simulink model "class_d_ff"  (R2024b)
settings: Solver=VariableStepAuto  StartTime=0.0  StopTime=5e-3  MaxStep=1e-8  RelTol=1e-9
undefined symbols (not defined in the file): gaussian
libraries: simulink x2
settings Model: SimulationMode=rapid-accelerator  Creator=Aaron  LastModifiedBy=Aaron
settings SolverCC: ShapePreserveControl=EnableAll  ZeroCrossAlgorithm=Adaptive

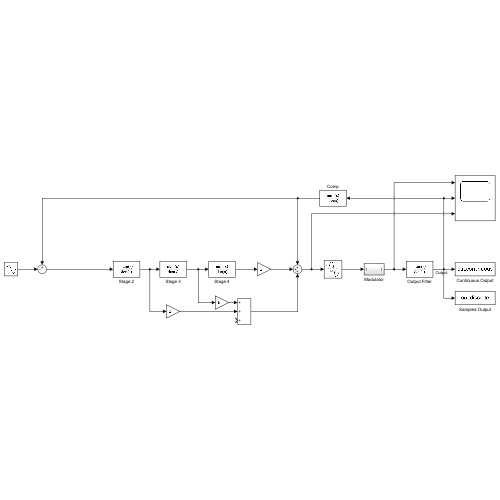
[thumbnail: Simulink's stored preview of the top-level diagram]
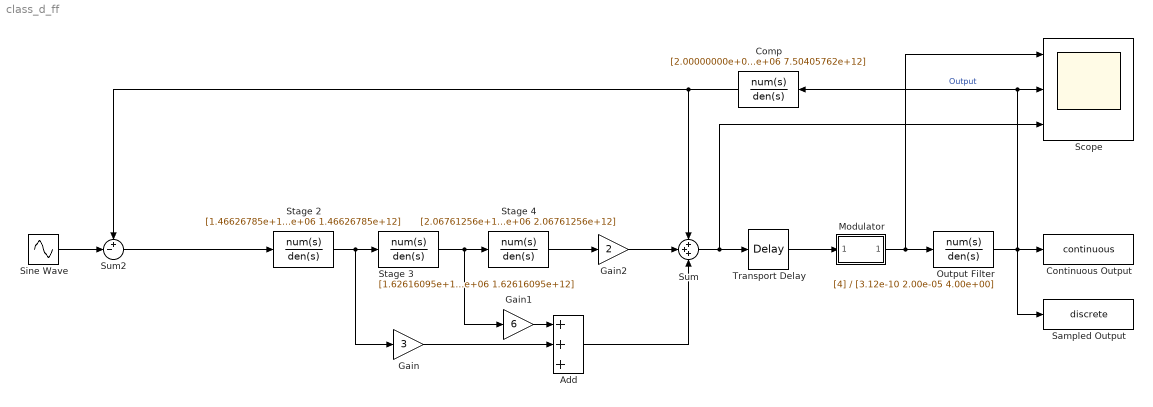
== system class_d_ff ==
  Add : Sum  Inputs=+++
  Comp : TransferFcn  Numerator=[2.00000000e+00 6.03185789e+06 4.54791371e+12]  Denominator=[1.00000000e+00 5.57946855e+06 7.50405762e+12]
  Continuous Output : ToWorkspace  VariableName=continuous  SaveFormat=Structure With Time  SampleTime=-1
  Gain : Gain  Gain=3
  Gain1 : Gain  Gain=6
  Gain2 : Gain  Gain=2
  Modulator : Subsystem
  Output Filter : TransferFcn  Numerator=[4]  Denominator=[3.12e-10 2.00e-05 4.00e+00]
  Sampled Output : ToWorkspace  VariableName=discrete  SampleTime=-1
  Scope : Scope  NumInputPorts=3
  Sine Wave : Sin  Amplitude=8  Frequency=2*pi*1e3  SampleTime=0
  Stage 2 : TransferFcn  Numerator=[1.46626785e+12]  Denominator=[1.00000000e+00 3.81089188e+06 1.46626785e+12]
  Stage 3 : TransferFcn  Numerator=[1.62616095e+12]  Denominator=[1.00000000e+00 3.52873517e+06 1.62616095e+12]
  Stage 4 : TransferFcn  Numerator=[2.06761256e+12]  Denominator=[1.00000000e+00 2.67955474e+06 2.06761256e+12]
  Sum : Sum  Inputs=+++
  Sum2 : Sum  Inputs=+-|
  Transport Delay : TransportDelay  DelayTime=140e-9
  wires:
  Transport Delay/1 -> Modulator/1(Input)
  Modulator/1(Output) -> Scope/1, Output Filter/1
  Output Filter/1 -> Sampled Output/1, Continuous Output/1, Scope/2, Comp/1  "Output"
  Sine Wave/1 -> Sum2/2
  Comp/1 -> Sum2/1, Sum/1
  Sum/1 -> Scope/3, Transport Delay/1
  Stage 4/1 -> Gain2/1
  Add/1 -> Sum/3
  Stage 3/1 -> Stage 4/1, Gain1/1
  Gain/1 -> Add/2
  Gain1/1 -> Add/1
  Gain2/1 -> Sum/2
  Stage 2/1 -> Gain/1, Stage 3/1
  Sum2/1 -> Stage 2/1

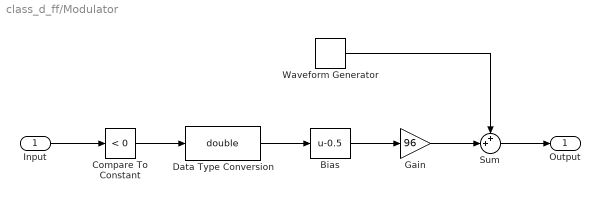
== system class_d_ff/Modulator ==
  Input : Inport
  Bias : Bias  Bias=-0.5  SaturateOnIntegerOverflow=off
  Compare To Constant : simulink/Logic and Bit Operations/Compare To Constant  relop=<  const=0  OutDataTypeStr=uint8
  Data Type Conversion : DataTypeConversion  OutDataTypeStr=double  SaturateOnIntegerOverflow=off  RndMeth=Floor
  Gain : Gain  Gain=96
  Sum : Sum  Inputs=++|
  Waveform Generator : simulink/Sources/Waveform Generator  OutMin=[]  OutMax=[]  OutDataTypeStr=double  SelectedSignal=1  Signals=gaussian('Variance',1e-1)  BlockNames=MultiportSwitch_ce802b024d02497  SampleTime=0.1
  Output : Outport
  wires:
  Input/1 -> Compare To Constant/1
  Data Type Conversion/1 -> Bias/1
  Compare To Constant/1 -> Data Type Conversion/1
  Bias/1 -> Gain/1
  Waveform Generator/1 -> Sum/1
  Gain/1 -> Sum/2
  Sum/1 -> Output/1
